simulink model "ChenEx3p3p3"  (R2014a)
settings: Solver=ode45  StartTime=0.0  StopTime=TSIM  RelTol=1e-3
values from neighbouring files (symbols this model uses):
  A = [ ... (first row only)    [chenEx3p3p3.m]
  B = [1 0 0;0 1 0; 0 0 1;0 0 0]    [chenEx3p3p3.m]
  F1 = [ ... (first row only)    [chenEx3p3p3.m]
  fa1 = 1    [chenEx3p3p3.m]
  fa2 = 0    [chenEx3p3p3.m]
  fa3 = 0    [chenEx3p3p3.m]
  ICH1 = eye(3)-C*H1    [chenEx3p3p3.m]
  K1 = [ ... (first row only)    [chenEx3p3p3.m]
  T1 = [ ... (first row only)    [chenEx3p3p3.m]
  u1Val = 34.632    [chenEx3p3p3.m]
  u2Val = 1641.6    [chenEx3p3p3.m]
  u3Val = 29980    [chenEx3p3p3.m]
  X0 = [0.3412;525.7;525.7;496.2]    [chenEx3p3p3.m]
settings Model: Creator=nazari.s  LastModifiedBy=samnazari
settings DebuggingCC: UnderspecifiedInitializationDetection=Classic

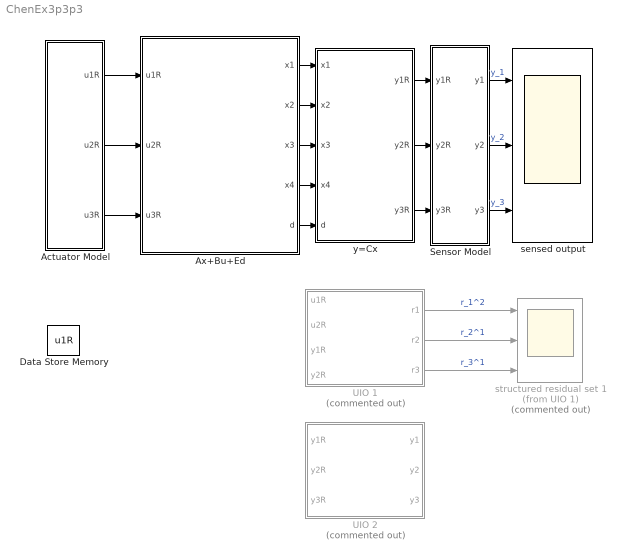
== system ChenEx3p3p3 ==
  Actuator Model : Subsystem
  Ax+Bu+Ed : Subsystem
  Data Store Memory : DataStoreMemory  DataStoreName=u1R  ReadBeforeWriteMsg=warning  WriteAfterWriteMsg=warning  WriteAfterReadMsg=warning
  Sensor Model : Subsystem
  UIO 1 : Subsystem  Commented=on
  UIO 2 : Subsystem  Commented=on
  sensed output : Scope  NumInputPorts=3
      settings: TimeRange=20  YMin=0~380~500  YMax=10~540~850
  structured residual set 1 (from UIO 1) : Scope  Commented=on  NumInputPorts=3
      settings: TimeRange=20  YMin=-1400~-1~-1  YMax=0~1~1
  y=Cx : Subsystem
  wires:
  Ax+Bu+Ed/1(x1) -> y=Cx/1(x1)
  Ax+Bu+Ed/2(x2) -> y=Cx/2(x2)
  Ax+Bu+Ed/3(x3) -> y=Cx/3(x3)
  Ax+Bu+Ed/4(x4) -> y=Cx/4(x4)
  Ax+Bu+Ed/5(d) -> y=Cx/5(d)
  Actuator Model/1(u1R) -> Ax+Bu+Ed/1(u1R)
  Actuator Model/2(u2R) -> Ax+Bu+Ed/2(u2R)
  Actuator Model/3(u3R) -> Ax+Bu+Ed/3(u3R)
  y=Cx/2(y2R) -> Sensor Model/2(y2R)
  y=Cx/3(y3R) -> Sensor Model/3(y3R)
  Sensor Model/1(y1) -> sensed output/1  "y_1"
  Sensor Model/2(y2) -> sensed output/2  "y_2"
  Sensor Model/3(y3) -> sensed output/3  "y_3"
  UIO 1/1(r1) -> structured residual set 1 (from UIO 1)/1  "r_1^2"
  UIO 1/2(r2) -> structured residual set 1 (from UIO 1)/2  "r_2^1"
  UIO 1/3("r3 ") -> structured residual set 1 (from UIO 1)/3  "r_3^1"
  y=Cx/1(y1R) -> Sensor Model/1(y1R)

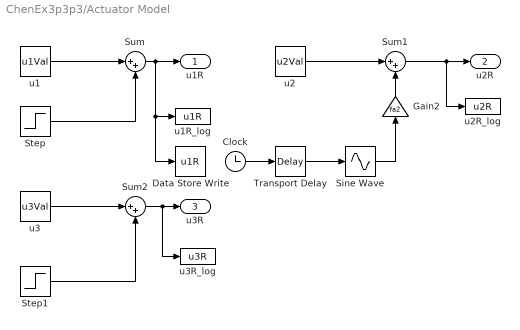
== system ChenEx3p3p3/Actuator Model ==
  Clock : Clock
  Data Store Write : DataStoreWrite  DataStoreName=u1R
  Gain2 : Gain  Gain=fa2
  Sine Wave : Sin  TimeSource=Use external signal  Amplitude=0.2*u2Val  Frequency=2  SampleTime=0
  Step : Step  Time=4  After=0.2*u1Val*fa1  SampleTime=0
  Step1 : Step  Time=4  After=-0.02*u3Val*fa3  SampleTime=0
  Sum : Sum  Inputs=|++
  Sum1 : Sum  Inputs=|++
  Sum2 : Sum  Inputs=|++
  Transport Delay : TransportDelay  DelayTime=4
  u1 : Constant  Value=u1Val
  u1R_log : ToWorkspace  VariableName=u1R  SampleTime=-1
      settings: Save2DSignal=2-D array (concatenate along first dimension)
  u2 : Constant  Value=u2Val
  u2R_log : ToWorkspace  VariableName=u2R  SampleTime=-1
      settings: Save2DSignal=2-D array (concatenate along first dimension)
  u3 : Constant  Value=u3Val
  u3R_log : ToWorkspace  VariableName=u3R  SampleTime=-1
      settings: Save2DSignal=2-D array (concatenate along first dimension)
  u1R : Outport
  u2R : Outport  Port=2
  u3R : Outport  Port=3
  wires:
  u2/1 -> Sum1/1
  Sum2/1 -> u3R_log/1, u3R/1
  u3/1 -> Sum2/1
  Sum/1 -> Data Store Write/1, u1R_log/1, u1R/1
  u1/1 -> Sum/1
  Sum1/1 -> u2R_log/1, u2R/1
  Gain2/1 -> Sum1/2
  Step/1 -> Sum/2
  Sine Wave/1 -> Gain2/1
  Transport Delay/1 -> Sine Wave/1
  Clock/1 -> Transport Delay/1
  Step1/1 -> Sum2/2

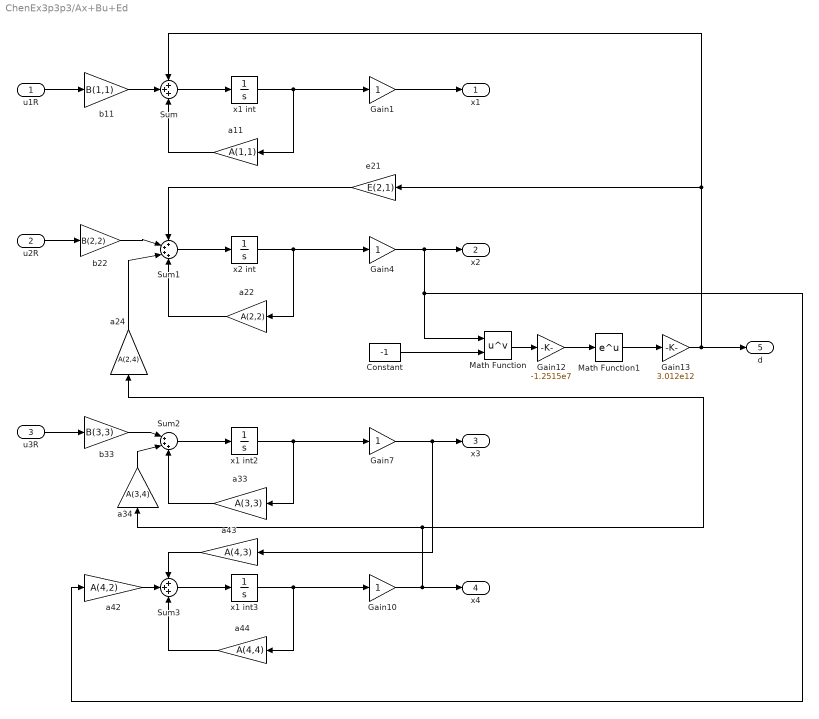
== system ChenEx3p3p3/Ax+Bu+Ed ==
  u1R : Inport
  u2R : Inport  Port=2
  u3R : Inport  Port=3
  Constant : Constant  Value=-1
  Gain{1,4,7,10} (4 alike) : Gain
  Gain12 : Gain  Gain=-1.2515e7
  Gain13 : Gain  Gain=3.012e12
  Math Function : Math  Operator=pow  SaturateOnIntegerOverflow=on
  Math Function1 : Math  SaturateOnIntegerOverflow=on
  Sum : Sum  Inputs=+++
  Sum1 : Sum  Inputs=++++
  Sum2 : Sum  Inputs=|+++
  Sum3 : Sum  Inputs=+++
  a11 : Gain  Gain=A(1,1)
  a22 : Gain  Gain=A(2,2)
  a24 : Gain  Gain=A(2,4)
  a33 : Gain  Gain=A(3,3)
  a34 : Gain  Gain=A(3,4)
  a42 : Gain  Gain=A(4,2)
  a43 : Gain  Gain=A(4,3)
  a44 : Gain  Gain=A(4,4)
  b11 : Gain  Gain=B(1,1)
  b22 : Gain  Gain=B(2,2)
  b33 : Gain  Gain=B(3,3)
  e21 : Gain  Gain=E(2,1)
  x1 int : Integrator  InitialCondition=X0(1,1)
  x1 int2 : Integrator  InitialCondition=X0(3,1)
  x1 int3 : Integrator  InitialCondition=X0(4,1)
  x2 int : Integrator  InitialCondition=X0(2,1)
  x1 : Outport
  x2 : Outport  Port=2
  x3 : Outport  Port=3
  x4 : Outport  Port=4
  d : Outport  Port=5
  wires:
  Sum3/1 -> x1 int3/1
  Gain10/1 -> x4/1, a24/1, a34/1
  Gain1/1 -> x1/1
  u1R/1 -> b11/1
  Sum/1 -> x1 int/1
  x2 int/1 -> Gain4/1, a22/1
  Sum1/1 -> x2 int/1
  Gain4/1 -> Math Function/1, a42/1, x2/1
  u2R/1 -> b22/1
  b33/1 -> Sum2/1
  a33/1 -> Sum2/3
  x1 int2/1 -> Gain7/1, a33/1
  Sum2/1 -> x1 int2/1
  Gain7/1 -> a43/1, x3/1
  u3R/1 -> b33/1
  x1 int3/1 -> Gain10/1, a44/1
  x1 int/1 -> Gain1/1, a11/1
  a11/1 -> Sum/3
  b11/1 -> Sum/2
  b22/1 -> Sum1/2
  a22/1 -> Sum1/4
  Constant/1 -> Math Function/2
  Math Function/1 -> Gain12/1
  Gain12/1 -> Math Function1/1
  Math Function1/1 -> Gain13/1
  Gain13/1 -> d/1, e21/1, Sum/1
  e21/1 -> Sum1/1
  a24/1 -> Sum1/3
  a34/1 -> Sum2/2
  a44/1 -> Sum3/3
  a43/1 -> Sum3/1
  a42/1 -> Sum3/2

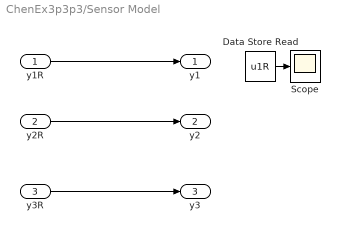
== system ChenEx3p3p3/Sensor Model ==
  y1R : Inport
  y2R : Inport  Port=2
  y3R : Inport  Port=3
  Data Store Read : DataStoreRead  DataStoreName=u1R
  Scope : Scope
      settings: SaveName=ScopeData2
  y1 : Outport
  y2 : Outport  Port=2
  y3 : Outport  Port=3
  wires:
  y1R/1 -> y1/1
  y2R/1 -> y2/1
  y3R/1 -> y3/1
  Data Store Read/1 -> Scope/1

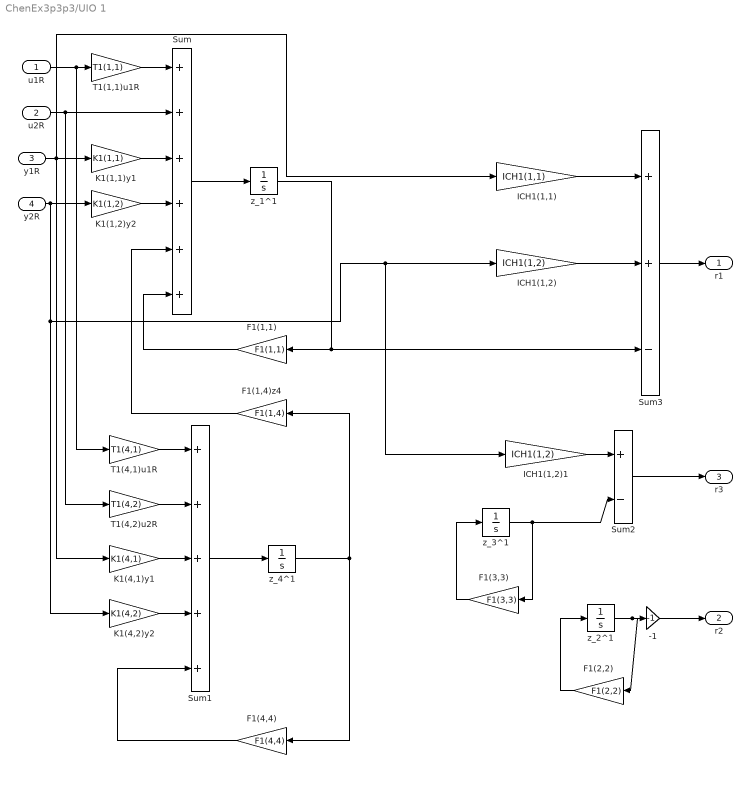
== system ChenEx3p3p3/UIO 1 ==
  u1R : Inport
  u2R : Inport  Port=2
  y1R : Inport  Port=3
  y2R : Inport  Port=4
  -1 : Gain  Gain=-1
  F1(1,1) : Gain  Gain=F1(1,1)
  F1(1,4)z4 : Gain  Gain=F1(1,4)
  F1(2,2) : Gain  Gain=F1(2,2)
  F1(3,3) : Gain  Gain=F1(3,3)
  F1(4,4) : Gain  Gain=F1(4,4)
  ICH1(1,1) : Gain  Gain=ICH1(1,1)
  ICH1(1,2) : Gain  Gain=ICH1(1,2)
  ICH1(1,2)1 : Gain  Gain=ICH1(1,2)
  K1(1,1)y1 : Gain  Gain=K1(1,1)
  K1(1,2)y2 : Gain  Gain=K1(1,2)
  K1(4,1)y1 : Gain  Gain=K1(4,1)
  K1(4,2)y2 : Gain  Gain=K1(4,2)
  Sum : Sum  Inputs=++++++
  Sum1 : Sum  Inputs=+++++
  Sum2 : Sum  Inputs=+-
  Sum3 : Sum  Inputs=++-
  T1(1,1)u1R : Gain  Gain=T1(1,1)
  T1(4,1)u1R : Gain  Gain=T1(4,1)
  T1(4,2)u2R : Gain  Gain=T1(4,2)
  z_1^1 : Integrator
  z_2^1 : Integrator
  z_3^1 : Integrator
  z_4^1 : Integrator
  r1 : Outport
  r2 : Outport  Port=2
  "r3 " : Outport  Port=3
  wires:
  z_1^1/1 -> F1(1,1)/1, Sum3/3
  Sum/1 -> z_1^1/1
  F1(1,1)/1 -> Sum/6
  F1(1,4)z4/1 -> Sum/5
  K1(1,2)y2/1 -> Sum/4
  K1(1,1)y1/1 -> Sum/3
  T1(1,1)u1R/1 -> Sum/1
  z_2^1/1 -> F1(2,2)/1, -1/1
  F1(2,2)/1 -> z_2^1/1
  z_3^1/1 -> Sum2/2, F1(3,3)/1
  F1(3,3)/1 -> z_3^1/1
  z_4^1/1 -> F1(4,4)/1, F1(1,4)z4/1
  Sum1/1 -> z_4^1/1
  F1(4,4)/1 -> Sum1/5
  K1(4,2)y2/1 -> Sum1/4
  K1(4,1)y1/1 -> Sum1/3
  T1(4,1)u1R/1 -> Sum1/1
  T1(4,2)u2R/1 -> Sum1/2
  ICH1(1,1)/1 -> Sum3/1
  ICH1(1,2)/1 -> Sum3/2
  Sum3/1 -> r1/1
  -1/1 -> r2/1
  y2R/1 -> ICH1(1,2)1/1, ICH1(1,2)/1, K1(4,2)y2/1, K1(1,2)y2/1
  ICH1(1,2)1/1 -> Sum2/1
  Sum2/1 -> "r3 "/1
  y1R/1 -> ICH1(1,1)/1, K1(4,1)y1/1, K1(1,1)y1/1
  u1R/1 -> T1(4,1)u1R/1, T1(1,1)u1R/1
  u2R/1 -> T1(4,2)u2R/1, Sum/2

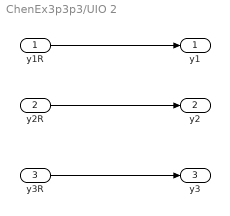
== system ChenEx3p3p3/UIO 2 ==
  y1R : Inport
  y2R : Inport  Port=2
  y3R : Inport  Port=3
  y1 : Outport
  y2 : Outport  Port=2
  y3 : Outport  Port=3
  wires:
  y1R/1 -> y1/1
  y2R/1 -> y2/1
  y3R/1 -> y3/1

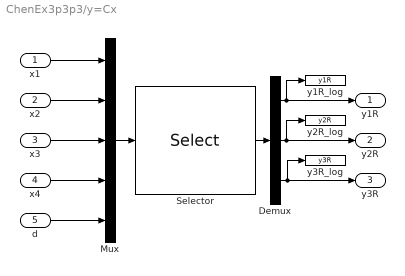
== system ChenEx3p3p3/y=Cx ==
  x1 : Inport
  x2 : Inport  Port=2
  x3 : Inport  Port=3
  x4 : Inport  Port=4
  d : Inport  Port=5
  Demux : Demux  Outputs=3
  Mux : Mux  Inputs=5
  Selector : Selector  InputPortWidth=5  Indices=[1 2 3]
  y1R_log : ToWorkspace  VariableName=y1R  SampleTime=-1
      settings: Save2DSignal=2-D array (concatenate along first dimension)
  y2R_log : ToWorkspace  VariableName=y2R  SampleTime=-1
      settings: Save2DSignal=2-D array (concatenate along first dimension)
  y3R_log : ToWorkspace  VariableName=y3R  SampleTime=-1
      settings: Save2DSignal=2-D array (concatenate along first dimension)
  y1R : Outport
  y2R : Outport  Port=2
  y3R : Outport  Port=3
  wires:
  x3/1 -> Mux/3
  x2/1 -> Mux/2
  x1/1 -> Mux/1
  x4/1 -> Mux/4
  Mux/1 -> Selector/1
  d/1 -> Mux/5
  Selector/1 -> Demux/1
  Demux/1 -> y1R/1, y1R_log/1
  Demux/3 -> y3R/1, y3R_log/1
  Demux/2 -> y2R/1, y2R_log/1
